simulink model "unrolled_pipelined_parallel"  (R2015b)
settings: Solver=FixedStepDiscrete  SolverMode=SingleTasking  StartTime=0.0  StopTime=10.0  RelTol=1e-3
undefined symbols (not defined in the file or in its folder): a, b
libraries: shlslibv1 x8781
(part 1 of 32)
settings Model: synDspstartup=OK  Creator=hchempat  LastModifiedBy=hchempat
settings DataIOCC: SaveOutput=off  SignalLogging=off  SaveTime=off
settings OptimizationCC: DefaultParameterBehavior=Inlined
settings DebuggingCC: AlgebraicLoopMsg=error  InheritedTsInSrcMsg=none

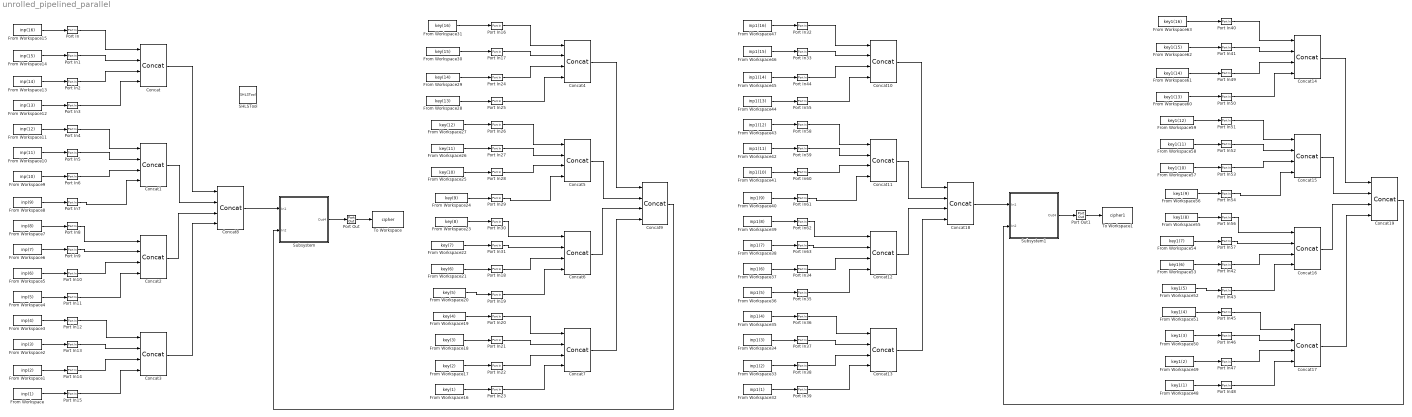
== system unrolled_pipelined_parallel ==
  Concat{,1..19} (20 alike) : shlslibv1/Signal Operations/Concat  syn_in_nb=4  syn_out_f=Automatic  syn_out_wl=16  syn_out_fl=8  syn_out_dt=signed  syn_en_se=off  synBlockType=primitive  synLatency=0  synBlockId=8
  From Workspace : FromWorkspace  VariableName=inp(1)
  From Workspace1 : FromWorkspace  VariableName=inp(2)
  From Workspace10 : FromWorkspace  VariableName=inp(11)
  From Workspace11 : FromWorkspace  VariableName=inp(12)
  From Workspace12 : FromWorkspace  VariableName=inp(13)
  From Workspace13 : FromWorkspace  VariableName=inp(14)
  From Workspace14 : FromWorkspace  VariableName=inp(15)
  From Workspace15 : FromWorkspace  VariableName=inp(16)
  From Workspace16 : FromWorkspace  VariableName=key(1)
  From Workspace17 : FromWorkspace  VariableName=key(2)
  From Workspace18 : FromWorkspace  VariableName=key(3)
  From Workspace19 : FromWorkspace  VariableName=key(4)
  From Workspace2 : FromWorkspace  VariableName=inp(3)
  From Workspace20 : FromWorkspace  VariableName=key(5)
  From Workspace21 : FromWorkspace  VariableName=key(6)
  From Workspace22 : FromWorkspace  VariableName=key(7)
  From Workspace23 : FromWorkspace  VariableName=key(8)
  From Workspace24 : FromWorkspace  VariableName=key(9)
  From Workspace25 : FromWorkspace  VariableName=key(10)
  From Workspace26 : FromWorkspace  VariableName=key(11)
  From Workspace27 : FromWorkspace  VariableName=key(12)
  From Workspace28 : FromWorkspace  VariableName=key(13)
  From Workspace29 : FromWorkspace  VariableName=key(14)
  From Workspace3 : FromWorkspace  VariableName=inp(4)
  From Workspace30 : FromWorkspace  VariableName=key(15)
  From Workspace31 : FromWorkspace  VariableName=key(16)
  From Workspace32 : FromWorkspace  VariableName=inp1(1)
  From Workspace33 : FromWorkspace  VariableName=inp1(2)
  From Workspace34 : FromWorkspace  VariableName=inp1(3)
  From Workspace35 : FromWorkspace  VariableName=inp1(4)
  From Workspace36 : FromWorkspace  VariableName=inp1(5)
  From Workspace37 : FromWorkspace  VariableName=inp1(6)
  From Workspace38 : FromWorkspace  VariableName=inp1(7)
  From Workspace39 : FromWorkspace  VariableName=inp1(8)
  From Workspace4 : FromWorkspace  VariableName=inp(5)
  From Workspace40 : FromWorkspace  VariableName=inp1(9)
  From Workspace41 : FromWorkspace  VariableName=inp1(10)
  From Workspace42 : FromWorkspace  VariableName=inp1(11)
  From Workspace43 : FromWorkspace  VariableName=inp1(12)
  From Workspace44 : FromWorkspace  VariableName=inp1(13)
  From Workspace45 : FromWorkspace  VariableName=inp1(14)
  From Workspace46 : FromWorkspace  VariableName=inp1(15)
  From Workspace47 : FromWorkspace  VariableName=inp1(16)
  From Workspace48 : FromWorkspace  VariableName=key1(1)
  From Workspace49 : FromWorkspace  VariableName=key1(2)
  From Workspace5 : FromWorkspace  VariableName=inp(6)
  From Workspace50 : FromWorkspace  VariableName=key1(3)
  From Workspace51 : FromWorkspace  VariableName=key1(4)
  From Workspace52 : FromWorkspace  VariableName=key1(5)
  From Workspace53 : FromWorkspace  VariableName=key1(6)
  From Workspace54 : FromWorkspace  VariableName=key1(7)
  From Workspace55 : FromWorkspace  VariableName=key1(8)
  From Workspace56 : FromWorkspace  VariableName=key1(9)
  From Workspace57 : FromWorkspace  VariableName=key1(10)
  From Workspace58 : FromWorkspace  VariableName=key1(11)
  From Workspace59 : FromWorkspace  VariableName=key1(12)
  From Workspace6 : FromWorkspace  VariableName=inp(7)
  From Workspace60 : FromWorkspace  VariableName=key1(13)
  From Workspace61 : FromWorkspace  VariableName=key1(14)
  From Workspace62 : FromWorkspace  VariableName=key1(15)
  From Workspace63 : FromWorkspace  VariableName=key1(16)
  From Workspace7 : FromWorkspace  VariableName=inp(8)
  From Workspace8 : FromWorkspace  VariableName=inp(9)
  From Workspace9 : FromWorkspace  VariableName=inp(10)
  Port In{,1..63} (64 alike) : shlslibv1/Ports & Subsystems/Port In  syn_out_wl=8  syn_out_fl=0  syn_out_dt=unsigned  syn_out_st=ts  syn_capture=on  syn_register=on  syn_out_sat=off  syn_out_rnd=on  synBlockType=port  synLatency=1  synBlockId=0
  Port Out : shlslibv1/Ports & Subsystems/Port Out  syn_capture=on  syn_register=on  synBlockType=port  synLatency=1  synBlockId=1
  Port Out1 : shlslibv1/Ports & Subsystems/Port Out  syn_capture=on  syn_register=on  synBlockType=port  synLatency=1  synBlockId=1
  SHLSTool : shlslibv1/SHLSTool  synBlockType=tool  syn_dsp_mode=FPGA
  Subsystem : Subsystem
  Subsystem1 : Subsystem
  To Workspace : ToWorkspace  VariableName=cipher  SaveFormat=Structure With Time  SampleTime=-1
  To Workspace1 : ToWorkspace  VariableName=cipher1  SaveFormat=Structure With Time  SampleTime=-1
  wires:
  From Workspace15/1 -> Port In/1
  From Workspace14/1 -> Port In1/1
  From Workspace12/1 -> Port In3/1
  From Workspace13/1 -> Port In2/1
  From Workspace11/1 -> Port In4/1
  From Workspace10/1 -> Port In5/1
  From Workspace9/1 -> Port In6/1
  From Workspace8/1 -> Port In7/1
  From Workspace7/1 -> Port In8/1
  From Workspace6/1 -> Port In9/1
  From Workspace5/1 -> Port In10/1
  From Workspace4/1 -> Port In11/1
  From Workspace3/1 -> Port In12/1
  From Workspace2/1 -> Port In13/1
  From Workspace1/1 -> Port In14/1
  From Workspace/1 -> Port In15/1
  Port In2/1 -> Concat/3
  Port In1/1 -> Concat/2
  Port In/1 -> Concat/1
  Port In3/1 -> Concat/4
  Port In6/1 -> Concat1/3
  Port In5/1 -> Concat1/2
  Port In4/1 -> Concat1/1
  Port In7/1 -> Concat1/4
  Port In10/1 -> Concat2/3
  Port In9/1 -> Concat2/2
  Port In8/1 -> Concat2/1
  Port In11/1 -> Concat2/4
  Port In14/1 -> Concat3/3
  Port In13/1 -> Concat3/2
  Port In15/1 -> Concat3/4
  Port In12/1 -> Concat3/1
  From Workspace22/1 -> Port In31/1
  From Workspace21/1 -> Port In18/1
  From Workspace20/1 -> Port In19/1
  From Workspace18/1 -> Port In21/1
  From Workspace17/1 -> Port In22/1
  From Workspace16/1 -> Port In23/1
  Port In24/1 -> Concat4/3
  Port In17/1 -> Concat4/2
  Port In16/1 -> Concat4/1
  Port In25/1 -> Concat4/4
  Port In28/1 -> Concat5/3
  Port In27/1 -> Concat5/2
  Port In26/1 -> Concat5/1
  Port In29/1 -> Concat5/4
  Port In18/1 -> Concat6/3
  Port In31/1 -> Concat6/2
  Port In30/1 -> Concat6/1
  Port In19/1 -> Concat6/4
  Port In22/1 -> Concat7/3
  Port In21/1 -> Concat7/2
  Port In23/1 -> Concat7/4
  Port In20/1 -> Concat7/1
  Concat/1 -> Concat8/1
  Concat1/1 -> Concat8/2
  Concat2/1 -> Concat8/3
  Concat3/1 -> Concat8/4
  Concat4/1 -> Concat9/1
  Concat5/1 -> Concat9/2
  Concat6/1 -> Concat9/3
  Concat7/1 -> Concat9/4
  Port Out/1 -> To Workspace/1
  Concat8/1 -> Subsystem/1(In1)
  Concat9/1 -> Subsystem/2(In2)
  Subsystem/1(Out4) -> Port Out/1
  From Workspace19/1 -> Port In20/1
  From Workspace23/1 -> Port In30/1
  From Workspace24/1 -> Port In29/1
  From Workspace25/1 -> Port In28/1
  From Workspace27/1 -> Port In26/1
  From Workspace28/1 -> Port In25/1
  From Workspace29/1 -> Port In24/1
  From Workspace30/1 -> Port In17/1
  From Workspace31/1 -> Port In16/1
  From Workspace26/1 -> Port In27/1
  From Workspace47/1 -> Port In32/1
  From Workspace46/1 -> Port In33/1
  From Workspace44/1 -> Port In55/1
  From Workspace45/1 -> Port In44/1
  From Workspace43/1 -> Port In58/1
  From Workspace42/1 -> Port In59/1
  From Workspace41/1 -> Port In60/1
  From Workspace40/1 -> Port In61/1
  From Workspace39/1 -> Port In62/1
  From Workspace38/1 -> Port In63/1
  From Workspace37/1 -> Port In34/1
  From Workspace36/1 -> Port In35/1
  From Workspace35/1 -> Port In36/1
  From Workspace34/1 -> Port In37/1
  From Workspace33/1 -> Port In38/1
  From Workspace32/1 -> Port In39/1
  Port In44/1 -> Concat10/3
  Port In33/1 -> Concat10/2
  Port In32/1 -> Concat10/1
  Port In55/1 -> Concat10/4
  Port In60/1 -> Concat11/3
  Port In59/1 -> Concat11/2
  Port In58/1 -> Concat11/1
  Port In61/1 -> Concat11/4
  Port In34/1 -> Concat12/3
  Port In63/1 -> Concat12/2
  Port In62/1 -> Concat12/1
  Port In35/1 -> Concat12/4
  Port In38/1 -> Concat13/3
  Port In37/1 -> Concat13/2
  Port In39/1 -> Concat13/4
  Port In36/1 -> Concat13/1
  From Workspace54/1 -> Port In57/1
  From Workspace53/1 -> Port In42/1
  From Workspace52/1 -> Port In43/1
  From Workspace50/1 -> Port In46/1
  From Workspace49/1 -> Port In47/1
  From Workspace48/1 -> Port In48/1
  Port In49/1 -> Concat14/3
  Port In41/1 -> Concat14/2
  Port In40/1 -> Concat14/1
  Port In50/1 -> Concat14/4
  Port In53/1 -> Concat15/3
  Port In52/1 -> Concat15/2
  Port In51/1 -> Concat15/1
  Port In54/1 -> Concat15/4
  Port In42/1 -> Concat16/3
  Port In57/1 -> Concat16/2
  Port In56/1 -> Concat16/1
  Port In43/1 -> Concat16/4
  Port In47/1 -> Concat17/3
  Port In46/1 -> Concat17/2
  Port In48/1 -> Concat17/4
  Port In45/1 -> Concat17/1
  Concat10/1 -> Concat18/1
  Concat11/1 -> Concat18/2
  Concat12/1 -> Concat18/3
  Concat13/1 -> Concat18/4
  Concat14/1 -> Concat19/1
  Concat15/1 -> Concat19/2
  Concat16/1 -> Concat19/3
  Concat17/1 -> Concat19/4
  Port Out1/1 -> To Workspace1/1
  Concat18/1 -> Subsystem1/1(In1)
  Concat19/1 -> Subsystem1/2(In2)
  Subsystem1/1(Out4) -> Port Out1/1
  From Workspace51/1 -> Port In45/1
  From Workspace55/1 -> Port In56/1
  From Workspace56/1 -> Port In54/1
  From Workspace57/1 -> Port In53/1
  From Workspace59/1 -> Port In51/1
  From Workspace60/1 -> Port In50/1
  From Workspace61/1 -> Port In49/1
  From Workspace62/1 -> Port In41/1
  From Workspace63/1 -> Port In40/1
  From Workspace58/1 -> Port In52/1

== system unrolled_pipelined_parallel/Subsystem ==
  In1 : Inport
  In2 : Inport  Port=2
  Concat : shlslibv1/Signal Operations/Concat  syn_in_nb=4  syn_out_f=Automatic  syn_out_wl=16  syn_out_fl=8  syn_out_dt=signed  syn_en_se=off  synBlockType=primitive  synLatency=0  synBlockId=8
  FINALROUND : Subsystem
  Register{1..50} (50 alike) : shlslibv1/Memories/Register  syn_delay_val=1  syn_rst_val=All zeros  syn_rst_vec=5  syn_rst_port=off  syn_en_port=off  synBlockType=custom  synLatency=1
  Subsystem : Subsystem
  Subsystem1 : Subsystem
  Subsystem2 : Subsystem
  Subsystem3 : Subsystem
  Subsystem4 : Subsystem
  Subsystem5 : Subsystem
  Subsystem6 : Subsystem
  Subsystem7 : Subsystem
  Subsystem8 : Subsystem
  Subsystem9 : Subsystem
  Out4 : Outport
  wires:
  FINALROUND/4(Out4) -> Concat/4
  FINALROUND/3(Out3) -> Concat/3
  FINALROUND/2(Out2) -> Concat/2
  FINALROUND/1(Out1) -> Concat/1
  In2/1 -> Register46/1, Subsystem/2(In2)
  In1/1 -> Subsystem/1(In1)
  Concat/1 -> Out4/1
  Subsystem1/5(Out5) -> Register5/1
  Register5/1 -> Subsystem2/5(In5)
  Subsystem1/2(Out2) -> Register2/1
  Subsystem1/3(Out3) -> Register3/1
  Subsystem1/4(Out4) -> Register4/1
  Subsystem1/1(Out1) -> Register1/1
  Register1/1 -> Subsystem2/1(In1)
  Register2/1 -> Subsystem2/2(In2)
  Register3/1 -> Subsystem2/3(In3)
  Register4/1 -> Subsystem2/4(In4)
  Subsystem2/5(Out5) -> Register10/1
  Subsystem2/2(Out2) -> Register7/1
  Subsystem2/3(Out3) -> Register8/1
  Subsystem2/4(Out4) -> Register9/1
  Subsystem2/1(Out1) -> Register6/1
  Register8/1 -> Subsystem3/3(In3)
  Register9/1 -> Subsystem3/4(In4)
  Register7/1 -> Subsystem3/2(In2)
  Register6/1 -> Subsystem3/1(In1)
  Register10/1 -> Subsystem3/5(In5)
  Subsystem3/5(Out5) -> Register11/1
  Subsystem3/2(Out2) -> Register13/1
  Subsystem3/3(Out3) -> Register14/1
  Subsystem3/4(Out4) -> Register15/1
  Subsystem3/1(Out1) -> Register12/1
  Register14/1 -> Subsystem4/3(In3)
  Register15/1 -> Subsystem4/4(In4)
  Register13/1 -> Subsystem4/2(In2)
  Register12/1 -> Subsystem4/1(In1)
  Register11/1 -> Subsystem4/5(In5)
  Subsystem4/5(Out5) -> Register16/1
  Subsystem4/2(Out2) -> Register18/1
  Subsystem4/3(Out3) -> Register19/1
  Subsystem4/4(Out4) -> Register20/1
  Subsystem4/1(Out1) -> Register17/1
  Register19/1 -> Subsystem5/3(In3)
  Register20/1 -> Subsystem5/4(In4)
  Register18/1 -> Subsystem5/2(In2)
  Register17/1 -> Subsystem5/1(In1)
  Register16/1 -> Subsystem5/5(In5)
  Subsystem5/5(Out5) -> Register21/1
  Subsystem5/2(Out2) -> Register23/1
  Subsystem5/3(Out3) -> Register24/1
  Subsystem5/4(Out4) -> Register25/1
  Subsystem5/1(Out1) -> Register22/1
  Register24/1 -> Subsystem6/3(In3)
  Register25/1 -> Subsystem6/4(In4)
  Register23/1 -> Subsystem6/2(In2)
  Register22/1 -> Subsystem6/1(In1)
  Register21/1 -> Subsystem6/5(In5)
  Subsystem6/5(Out5) -> Register26/1
  Subsystem6/2(Out2) -> Register28/1
  Subsystem6/3(Out3) -> Register29/1
  Subsystem6/4(Out4) -> Register30/1
  Subsystem6/1(Out1) -> Register27/1
  Register29/1 -> Subsystem7/3(In3)
  Register30/1 -> Subsystem7/4(In4)
  Register28/1 -> Subsystem7/2(In2)
  Register27/1 -> Subsystem7/1(In1)
  Register26/1 -> Subsystem7/5(In5)
  Subsystem7/5(Out5) -> Register31/1
  Subsystem7/2(Out2) -> Register33/1
  Subsystem7/3(Out3) -> Register34/1
  Subsystem7/4(Out4) -> Register35/1
  Subsystem7/1(Out1) -> Register32/1
  Register34/1 -> Subsystem8/3(In3)
  Register35/1 -> Subsystem8/4(In4)
  Register33/1 -> Subsystem8/2(In2)
  Register32/1 -> Subsystem8/1(In1)
  Register31/1 -> Subsystem8/5(In5)
  Subsystem8/5(Out5) -> Register36/1
  Subsystem8/2(Out2) -> Register38/1
  Subsystem8/3(Out3) -> Register39/1
  Subsystem8/4(Out4) -> Register40/1
  Subsystem8/1(Out1) -> Register37/1
  Register39/1 -> Subsystem9/3(In3)
  Register40/1 -> Subsystem9/4(In4)
  Register38/1 -> Subsystem9/2(In2)
  Register37/1 -> Subsystem9/1(In1)
  Register36/1 -> Subsystem9/5(In5)
  Subsystem9/5(Out5) -> Register41/1
  Subsystem9/2(Out2) -> Register43/1
  Subsystem9/3(Out3) -> Register44/1
  Subsystem9/4(Out4) -> Register45/1
  Subsystem9/1(Out1) -> Register42/1
  Register44/1 -> FINALROUND/3(In3)
  Register45/1 -> FINALROUND/4(In4)
  Register43/1 -> FINALROUND/2(In2)
  Register42/1 -> FINALROUND/1(In1)
  Register41/1 -> FINALROUND/5(In5)
  Register46/1 -> Subsystem1/5(In5)
  Subsystem/4(Out4) -> Register47/1
  Register47/1 -> Subsystem1/4(In4)
  Subsystem/1(Out1) -> Register50/1
  Register50/1 -> Subsystem1/1(In1)
  Subsystem/2(Out2) -> Register49/1
  Register49/1 -> Subsystem1/2(In2)
  Subsystem/3(Out3) -> Register48/1
  Register48/1 -> Subsystem1/3(In3)

== system unrolled_pipelined_parallel/Subsystem1 ==
  In1 : Inport
  In2 : Inport  Port=2
  Concat : shlslibv1/Signal Operations/Concat  syn_in_nb=4  syn_out_f=Automatic  syn_out_wl=16  syn_out_fl=8  syn_out_dt=signed  syn_en_se=off  synBlockType=primitive  synLatency=0  synBlockId=8
  FINALROUND : Subsystem
  Register{1..50} (50 alike) : shlslibv1/Memories/Register  syn_delay_val=1  syn_rst_val=All zeros  syn_rst_vec=5  syn_rst_port=off  syn_en_port=off  synBlockType=custom  synLatency=1
  Subsystem : Subsystem
  Subsystem1 : Subsystem
  Subsystem2 : Subsystem
  Subsystem3 : Subsystem
  Subsystem4 : Subsystem
  Subsystem5 : Subsystem
  Subsystem6 : Subsystem
  Subsystem7 : Subsystem
  Subsystem8 : Subsystem
  Subsystem9 : Subsystem
  Out4 : Outport
  wires:
  FINALROUND/4(Out4) -> Concat/4
  FINALROUND/3(Out3) -> Concat/3
  FINALROUND/2(Out2) -> Concat/2
  FINALROUND/1(Out1) -> Concat/1
  In2/1 -> Register46/1, Subsystem/2(In2)
  In1/1 -> Subsystem/1(In1)
  Concat/1 -> Out4/1
  Subsystem1/5(Out5) -> Register5/1
  Register5/1 -> Subsystem2/5(In5)
  Subsystem1/2(Out2) -> Register2/1
  Subsystem1/3(Out3) -> Register3/1
  Subsystem1/4(Out4) -> Register4/1
  Subsystem1/1(Out1) -> Register1/1
  Register1/1 -> Subsystem2/1(In1)
  Register2/1 -> Subsystem2/2(In2)
  Register3/1 -> Subsystem2/3(In3)
  Register4/1 -> Subsystem2/4(In4)
  Subsystem2/5(Out5) -> Register10/1
  Subsystem2/2(Out2) -> Register7/1
  Subsystem2/3(Out3) -> Register8/1
  Subsystem2/4(Out4) -> Register9/1
  Subsystem2/1(Out1) -> Register6/1
  Register8/1 -> Subsystem3/3(In3)
  Register9/1 -> Subsystem3/4(In4)
  Register7/1 -> Subsystem3/2(In2)
  Register6/1 -> Subsystem3/1(In1)
  Register10/1 -> Subsystem3/5(In5)
  Subsystem3/5(Out5) -> Register11/1
  Subsystem3/2(Out2) -> Register13/1
  Subsystem3/3(Out3) -> Register14/1
  Subsystem3/4(Out4) -> Register15/1
  Subsystem3/1(Out1) -> Register12/1
  Register14/1 -> Subsystem4/3(In3)
  Register15/1 -> Subsystem4/4(In4)
  Register13/1 -> Subsystem4/2(In2)
  Register12/1 -> Subsystem4/1(In1)
  Register11/1 -> Subsystem4/5(In5)
  Subsystem4/5(Out5) -> Register16/1
  Subsystem4/2(Out2) -> Register18/1
  Subsystem4/3(Out3) -> Register19/1
  Subsystem4/4(Out4) -> Register20/1
  Subsystem4/1(Out1) -> Register17/1
  Register19/1 -> Subsystem5/3(In3)
  Register20/1 -> Subsystem5/4(In4)
  Register18/1 -> Subsystem5/2(In2)
  Register17/1 -> Subsystem5/1(In1)
  Register16/1 -> Subsystem5/5(In5)
  Subsystem5/5(Out5) -> Register21/1
  Subsystem5/2(Out2) -> Register23/1
  Subsystem5/3(Out3) -> Register24/1
  Subsystem5/4(Out4) -> Register25/1
  Subsystem5/1(Out1) -> Register22/1
  Register24/1 -> Subsystem6/3(In3)
  Register25/1 -> Subsystem6/4(In4)
  Register23/1 -> Subsystem6/2(In2)
  Register22/1 -> Subsystem6/1(In1)
  Register21/1 -> Subsystem6/5(In5)
  Subsystem6/5(Out5) -> Register26/1
  Subsystem6/2(Out2) -> Register28/1
  Subsystem6/3(Out3) -> Register29/1
  Subsystem6/4(Out4) -> Register30/1
  Subsystem6/1(Out1) -> Register27/1
  Register29/1 -> Subsystem7/3(In3)
  Register30/1 -> Subsystem7/4(In4)
  Register28/1 -> Subsystem7/2(In2)
  Register27/1 -> Subsystem7/1(In1)
  Register26/1 -> Subsystem7/5(In5)
  Subsystem7/5(Out5) -> Register31/1
  Subsystem7/2(Out2) -> Register33/1
  Subsystem7/3(Out3) -> Register34/1
  Subsystem7/4(Out4) -> Register35/1
  Subsystem7/1(Out1) -> Register32/1
  Register34/1 -> Subsystem8/3(In3)
  Register35/1 -> Subsystem8/4(In4)
  Register33/1 -> Subsystem8/2(In2)
  Register32/1 -> Subsystem8/1(In1)
  Register31/1 -> Subsystem8/5(In5)
  Subsystem8/5(Out5) -> Register36/1
  Subsystem8/2(Out2) -> Register38/1
  Subsystem8/3(Out3) -> Register39/1
  Subsystem8/4(Out4) -> Register40/1
  Subsystem8/1(Out1) -> Register37/1
  Register39/1 -> Subsystem9/3(In3)
  Register40/1 -> Subsystem9/4(In4)
  Register38/1 -> Subsystem9/2(In2)
  Register37/1 -> Subsystem9/1(In1)
  Register36/1 -> Subsystem9/5(In5)
  Subsystem9/5(Out5) -> Register41/1
  Subsystem9/2(Out2) -> Register43/1
  Subsystem9/3(Out3) -> Register44/1
  Subsystem9/4(Out4) -> Register45/1
  Subsystem9/1(Out1) -> Register42/1
  Register44/1 -> FINALROUND/3(In3)
  Register45/1 -> FINALROUND/4(In4)
  Register43/1 -> FINALROUND/2(In2)
  Register42/1 -> FINALROUND/1(In1)
  Register41/1 -> FINALROUND/5(In5)
  Register46/1 -> Subsystem1/5(In5)
  Subsystem/4(Out4) -> Register47/1
  Register47/1 -> Subsystem1/4(In4)
  Subsystem/1(Out1) -> Register50/1
  Register50/1 -> Subsystem1/1(In1)
  Subsystem/2(Out2) -> Register49/1
  Register49/1 -> Subsystem1/2(In2)
  Subsystem/3(Out3) -> Register48/1
  Register48/1 -> Subsystem1/3(In3)

== system unrolled_pipelined_parallel/Subsystem/FINALROUND ==
  In1 : Inport
  In2 : Inport  Port=2
  In3 : Inport  Port=3
  In4 : Inport  Port=4
  In5 : Inport  Port=5
  ADD ROUND KEY : Subsystem
  KEYEXPANSION : Subsystem
  SB_rs_MIX_COLUMN : Subsystem
  Out1 : Outport
  Out2 : Outport  Port=2
  Out3 : Outport  Port=3
  Out4 : Outport  Port=4
  wires:
  SB_rs_MIX_COLUMN/1(Out1) -> ADD ROUND KEY/1(In1)
  KEYEXPANSION/1(Out1) -> ADD ROUND KEY/2(In2)
  In1/1 -> SB_rs_MIX_COLUMN/1(In1)
  In2/1 -> SB_rs_MIX_COLUMN/2(In2)
  In3/1 -> SB_rs_MIX_COLUMN/3(In3)
  In4/1 -> SB_rs_MIX_COLUMN/4(In4)
  In5/1 -> KEYEXPANSION/1(In1)
  ADD ROUND KEY/1(Out1) -> Out1/1
  ADD ROUND KEY/2(Out2) -> Out2/1
  ADD ROUND KEY/3(Out3) -> Out3/1
  ADD ROUND KEY/4(Out4) -> Out4/1

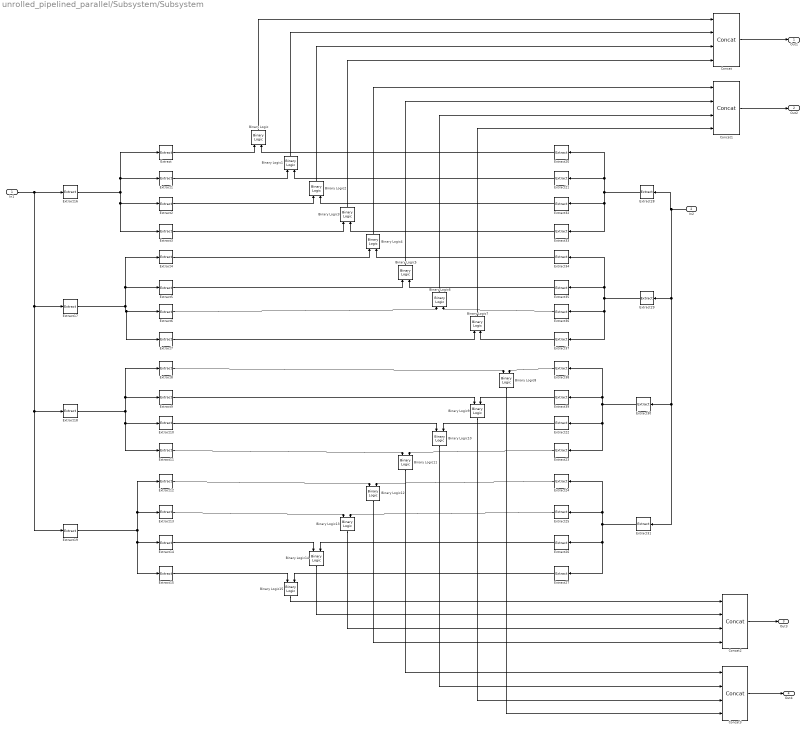
== system unrolled_pipelined_parallel/Subsystem/Subsystem ==
  In1 : Inport
  In2 : Inport  Port=2
  Binary Logic{,1..15} (16 alike) : shlslibv1/Math Functions/Binary Logic  syn_binlog_exp=a^b  synBlockType=primitive  synLatency=0  synBlockId=13
  Concat{,1..3} (4 alike) : shlslibv1/Signal Operations/Concat  syn_in_nb=4  syn_out_f=Automatic  syn_out_wl=16  syn_out_fl=8  syn_out_dt=signed  syn_en_se=off  synBlockType=primitive  synLatency=0  synBlockId=8
  Extract{,4,8,12,20,24,34,38} (8 alike) : shlslibv1/Signal Operations/Extract  syn_extract_vec=[24:31]  synBlockType=primitive  synLatency=0  synBlockId=17
  Extract{1,5,9,13,21,25,35,39} (8 alike) : shlslibv1/Signal Operations/Extract  syn_extract_vec=[16:23]  synBlockType=primitive  synLatency=0  synBlockId=17
  Extract{2,6,10,14,22,26,32,36} (8 alike) : shlslibv1/Signal Operations/Extract  syn_extract_vec=[8:15]  synBlockType=primitive  synLatency=0  synBlockId=17
  Extract{3,7,11,15,23,27,33,37} (8 alike) : shlslibv1/Signal Operations/Extract  syn_extract_vec=[0:7]  synBlockType=primitive  synLatency=0  synBlockId=17
  Extract16 : shlslibv1/Signal Operations/Extract  syn_extract_vec=[96:127]  synBlockType=primitive  synLatency=0  synBlockId=17
  Extract17 : shlslibv1/Signal Operations/Extract  syn_extract_vec=[64:95]  synBlockType=primitive  synLatency=0  synBlockId=17
  Extract18 : shlslibv1/Signal Operations/Extract  syn_extract_vec=[32:63]  synBlockType=primitive  synLatency=0  synBlockId=17
  Extract19 : shlslibv1/Signal Operations/Extract  syn_extract_vec=[0:31]  synBlockType=primitive  synLatency=0  synBlockId=17
  Extract28 : shlslibv1/Signal Operations/Extract  syn_extract_vec=[96:127]  synBlockType=primitive  synLatency=0  synBlockId=17
  Extract29 : shlslibv1/Signal Operations/Extract  syn_extract_vec=[64:95]  synBlockType=primitive  synLatency=0  synBlockId=17
  Extract30 : shlslibv1/Signal Operations/Extract  syn_extract_vec=[32:63]  synBlockType=primitive  synLatency=0  synBlockId=17
  Extract31 : shlslibv1/Signal Operations/Extract  syn_extract_vec=[0:31]  synBlockType=primitive  synLatency=0  synBlockId=17
  Out1 : Outport
  Out2 : Outport  Port=2
  Out3 : Outport  Port=3
  Out4 : Outport  Port=4
  wires:
  Extract16/1 -> Extract/1, Extract1/1, Extract2/1, Extract3/1
  Extract17/1 -> Extract6/1, Extract7/1, Extract4/1, Extract5/1
  Extract18/1 -> Extract9/1, Extract8/1, Extract10/1, Extract11/1
  Extract19/1 -> Extract12/1, Extract13/1, Extract15/1, Extract14/1
  In1/1 -> Extract19/1, Extract18/1, Extract17/1, Extract16/1
  In2/1 -> Extract31/1, Extract30/1, Extract29/1, Extract28/1
  Extract28/1 -> Extract21/1, Extract20/1, Extract33/1, Extract32/1
  Extract29/1 -> Extract35/1, Extract34/1, Extract36/1, Extract37/1
  Extract30/1 -> Extract23/1, Extract22/1, Extract38/1, Extract39/1
  Extract31/1 -> Extract24/1, Extract25/1, Extract27/1, Extract26/1
  Extract/1 -> Binary Logic/1
  Extract20/1 -> Binary Logic/2
  Extract1/1 -> Binary Logic1/1
  Extract21/1 -> Binary Logic1/2
  Extract2/1 -> Binary Logic2/1
  Extract32/1 -> Binary Logic2/2
  Extract3/1 -> Binary Logic3/1
  Extract33/1 -> Binary Logic3/2
  Extract4/1 -> Binary Logic4/1
  Extract34/1 -> Binary Logic4/2
  Extract5/1 -> Binary Logic5/1
  Extract35/1 -> Binary Logic5/2
  Extract6/1 -> Binary Logic6/1
  Extract36/1 -> Binary Logic6/2
  Extract7/1 -> Binary Logic7/1
  Extract37/1 -> Binary Logic7/2
  Extract8/1 -> Binary Logic8/1
  Extract38/1 -> Binary Logic8/2
  Extract9/1 -> Binary Logic9/1
  Extract39/1 -> Binary Logic9/2
  Extract22/1 -> Binary Logic10/2
  Extract10/1 -> Binary Logic10/1
  Extract23/1 -> Binary Logic11/2
  Extract11/1 -> Binary Logic11/1
  Extract12/1 -> Binary Logic12/1
  Extract24/1 -> Binary Logic12/2
  Extract13/1 -> Binary Logic13/1
  Extract25/1 -> Binary Logic13/2
  Extract14/1 -> Binary Logic14/1
  Extract26/1 -> Binary Logic14/2
  Extract15/1 -> Binary Logic15/1
  Extract27/1 -> Binary Logic15/2
  Binary Logic7/1 -> Concat1/4
  Binary Logic6/1 -> Concat1/3
  Binary Logic5/1 -> Concat1/2
  Binary Logic4/1 -> Concat1/1
  Binary Logic3/1 -> Concat/4
  Binary Logic2/1 -> Concat/3
  Binary Logic1/1 -> Concat/2
  Binary Logic/1 -> Concat/1
  Binary Logic15/1 -> Concat2/1
  Binary Logic14/1 -> Concat2/2
  Binary Logic13/1 -> Concat2/3
  Binary Logic12/1 -> Concat2/4
  Binary Logic11/1 -> Concat3/1
  Binary Logic10/1 -> Concat3/2
  Binary Logic9/1 -> Concat3/3
  Binary Logic8/1 -> Concat3/4
  Concat/1 -> Out1/1
  Concat1/1 -> Out2/1
  Concat2/1 -> Out3/1
  Concat3/1 -> Out4/1

== system unrolled_pipelined_parallel/Subsystem/Subsystem1 ==
  In1 : Inport
  In2 : Inport  Port=2
  In3 : Inport  Port=3
  In4 : Inport  Port=4
  In5 : Inport  Port=5
  ADD ROUND KEY : Subsystem
  KEYEXPANSION : Subsystem
  SB_rs_MIX_COLUMN : Subsystem
  Out1 : Outport
  Out2 : Outport  Port=2
  Out3 : Outport  Port=3
  Out4 : Outport  Port=4
  Out5 : Outport  Port=5
  wires:
  SB_rs_MIX_COLUMN/1(Out1) -> ADD ROUND KEY/1(In1)
  KEYEXPANSION/1(Out1) -> Out5/1, ADD ROUND KEY/2(In2)
  In1/1 -> SB_rs_MIX_COLUMN/1(In1)
  In2/1 -> SB_rs_MIX_COLUMN/2(In2)
  In3/1 -> SB_rs_MIX_COLUMN/3(In3)
  In4/1 -> SB_rs_MIX_COLUMN/4(In4)
  In5/1 -> KEYEXPANSION/1(In1)
  ADD ROUND KEY/1(Out1) -> Out1/1
  ADD ROUND KEY/2(Out2) -> Out2/1
  ADD ROUND KEY/3(Out3) -> Out3/1
  ADD ROUND KEY/4(Out4) -> Out4/1

== system unrolled_pipelined_parallel/Subsystem/Subsystem2 ==
  In1 : Inport
  In2 : Inport  Port=2
  In3 : Inport  Port=3
  In4 : Inport  Port=4
  In5 : Inport  Port=5
  ADD ROUND KEY : Subsystem
  KEYEXPANSION : Subsystem
  SB_rs_MIX_COLUMN : Subsystem
  Out1 : Outport
  Out2 : Outport  Port=2
  Out3 : Outport  Port=3
  Out4 : Outport  Port=4
  Out5 : Outport  Port=5
  wires:
  SB_rs_MIX_COLUMN/1(Out1) -> ADD ROUND KEY/1(In1)
  KEYEXPANSION/1(Out1) -> Out5/1, ADD ROUND KEY/2(In2)
  In1/1 -> SB_rs_MIX_COLUMN/1(In1)
  In2/1 -> SB_rs_MIX_COLUMN/2(In2)
  In3/1 -> SB_rs_MIX_COLUMN/3(In3)
  In4/1 -> SB_rs_MIX_COLUMN/4(In4)
  In5/1 -> KEYEXPANSION/1(In1)
  ADD ROUND KEY/1(Out1) -> Out1/1
  ADD ROUND KEY/2(Out2) -> Out2/1
  ADD ROUND KEY/3(Out3) -> Out3/1
  ADD ROUND KEY/4(Out4) -> Out4/1

== system unrolled_pipelined_parallel/Subsystem/Subsystem3 ==
  In1 : Inport
  In2 : Inport  Port=2
  In3 : Inport  Port=3
  In4 : Inport  Port=4
  In5 : Inport  Port=5
  ADD ROUND KEY : Subsystem
  KEYEXPANSION : Subsystem
  SB_rs_MIX_COLUMN : Subsystem
  Out1 : Outport
  Out2 : Outport  Port=2
  Out3 : Outport  Port=3
  Out4 : Outport  Port=4
  Out5 : Outport  Port=5
  wires:
  SB_rs_MIX_COLUMN/1(Out1) -> ADD ROUND KEY/1(In1)
  KEYEXPANSION/1(Out1) -> Out5/1, ADD ROUND KEY/2(In2)
  In1/1 -> SB_rs_MIX_COLUMN/1(In1)
  In2/1 -> SB_rs_MIX_COLUMN/2(In2)
  In3/1 -> SB_rs_MIX_COLUMN/3(In3)
  In4/1 -> SB_rs_MIX_COLUMN/4(In4)
  In5/1 -> KEYEXPANSION/1(In1)
  ADD ROUND KEY/1(Out1) -> Out1/1
  ADD ROUND KEY/2(Out2) -> Out2/1
  ADD ROUND KEY/3(Out3) -> Out3/1
  ADD ROUND KEY/4(Out4) -> Out4/1

== system unrolled_pipelined_parallel/Subsystem/Subsystem4 ==
  In1 : Inport
  In2 : Inport  Port=2
  In3 : Inport  Port=3
  In4 : Inport  Port=4
  In5 : Inport  Port=5
  ADD ROUND KEY : Subsystem
  KEYEXPANSION : Subsystem
  SB_rs_MIX_COLUMN : Subsystem
  Out1 : Outport
  Out2 : Outport  Port=2
  Out3 : Outport  Port=3
  Out4 : Outport  Port=4
  Out5 : Outport  Port=5
  wires:
  SB_rs_MIX_COLUMN/1(Out1) -> ADD ROUND KEY/1(In1)
  KEYEXPANSION/1(Out1) -> Out5/1, ADD ROUND KEY/2(In2)
  In1/1 -> SB_rs_MIX_COLUMN/1(In1)
  In2/1 -> SB_rs_MIX_COLUMN/2(In2)
  In3/1 -> SB_rs_MIX_COLUMN/3(In3)
  In4/1 -> SB_rs_MIX_COLUMN/4(In4)
  In5/1 -> KEYEXPANSION/1(In1)
  ADD ROUND KEY/1(Out1) -> Out1/1
  ADD ROUND KEY/2(Out2) -> Out2/1
  ADD ROUND KEY/3(Out3) -> Out3/1
  ADD ROUND KEY/4(Out4) -> Out4/1

== system unrolled_pipelined_parallel/Subsystem/Subsystem5 ==
  In1 : Inport
  In2 : Inport  Port=2
  In3 : Inport  Port=3
  In4 : Inport  Port=4
  In5 : Inport  Port=5
  ADD ROUND KEY : Subsystem
  KEYEXPANSION : Subsystem
  SB_rs_MIX_COLUMN : Subsystem
  Out1 : Outport
  Out2 : Outport  Port=2
  Out3 : Outport  Port=3
  Out4 : Outport  Port=4
  Out5 : Outport  Port=5
  wires:
  SB_rs_MIX_COLUMN/1(Out1) -> ADD ROUND KEY/1(In1)
  KEYEXPANSION/1(Out1) -> Out5/1, ADD ROUND KEY/2(In2)
  In1/1 -> SB_rs_MIX_COLUMN/1(In1)
  In2/1 -> SB_rs_MIX_COLUMN/2(In2)
  In3/1 -> SB_rs_MIX_COLUMN/3(In3)
  In4/1 -> SB_rs_MIX_COLUMN/4(In4)
  In5/1 -> KEYEXPANSION/1(In1)
  ADD ROUND KEY/1(Out1) -> Out1/1
  ADD ROUND KEY/2(Out2) -> Out2/1
  ADD ROUND KEY/3(Out3) -> Out3/1
  ADD ROUND KEY/4(Out4) -> Out4/1

== system unrolled_pipelined_parallel/Subsystem/Subsystem6 ==
  In1 : Inport
  In2 : Inport  Port=2
  In3 : Inport  Port=3
  In4 : Inport  Port=4
  In5 : Inport  Port=5
  ADD ROUND KEY : Subsystem
  KEYEXPANSION : Subsystem
  SB_rs_MIX_COLUMN : Subsystem
  Out1 : Outport
  Out2 : Outport  Port=2
  Out3 : Outport  Port=3
  Out4 : Outport  Port=4
  Out5 : Outport  Port=5
  wires:
  SB_rs_MIX_COLUMN/1(Out1) -> ADD ROUND KEY/1(In1)
  KEYEXPANSION/1(Out1) -> Out5/1, ADD ROUND KEY/2(In2)
  In1/1 -> SB_rs_MIX_COLUMN/1(In1)
  In2/1 -> SB_rs_MIX_COLUMN/2(In2)
  In3/1 -> SB_rs_MIX_COLUMN/3(In3)
  In4/1 -> SB_rs_MIX_COLUMN/4(In4)
  In5/1 -> KEYEXPANSION/1(In1)
  ADD ROUND KEY/1(Out1) -> Out1/1
  ADD ROUND KEY/2(Out2) -> Out2/1
  ADD ROUND KEY/3(Out3) -> Out3/1
  ADD ROUND KEY/4(Out4) -> Out4/1

== system unrolled_pipelined_parallel/Subsystem/Subsystem7 ==
  In1 : Inport
  In2 : Inport  Port=2
  In3 : Inport  Port=3
  In4 : Inport  Port=4
  In5 : Inport  Port=5
  ADD ROUND KEY : Subsystem
  KEYEXPANSION : Subsystem
  SB_rs_MIX_COLUMN : Subsystem
  Out1 : Outport
  Out2 : Outport  Port=2
  Out3 : Outport  Port=3
  Out4 : Outport  Port=4
  Out5 : Outport  Port=5
  wires:
  SB_rs_MIX_COLUMN/1(Out1) -> ADD ROUND KEY/1(In1)
  KEYEXPANSION/1(Out1) -> Out5/1, ADD ROUND KEY/2(In2)
  In1/1 -> SB_rs_MIX_COLUMN/1(In1)
  In2/1 -> SB_rs_MIX_COLUMN/2(In2)
  In3/1 -> SB_rs_MIX_COLUMN/3(In3)
  In4/1 -> SB_rs_MIX_COLUMN/4(In4)
  In5/1 -> KEYEXPANSION/1(In1)
  ADD ROUND KEY/1(Out1) -> Out1/1
  ADD ROUND KEY/2(Out2) -> Out2/1
  ADD ROUND KEY/3(Out3) -> Out3/1
  ADD ROUND KEY/4(Out4) -> Out4/1

== system unrolled_pipelined_parallel/Subsystem/Subsystem8 ==
  In1 : Inport
  In2 : Inport  Port=2
  In3 : Inport  Port=3
  In4 : Inport  Port=4
  In5 : Inport  Port=5
  ADD ROUND KEY : Subsystem
  KEYEXPANSION : Subsystem
  SB_rs_MIX_COLUMN : Subsystem
  Out1 : Outport
  Out2 : Outport  Port=2
  Out3 : Outport  Port=3
  Out4 : Outport  Port=4
  Out5 : Outport  Port=5
  wires:
  SB_rs_MIX_COLUMN/1(Out1) -> ADD ROUND KEY/1(In1)
  KEYEXPANSION/1(Out1) -> Out5/1, ADD ROUND KEY/2(In2)
  In1/1 -> SB_rs_MIX_COLUMN/1(In1)
  In2/1 -> SB_rs_MIX_COLUMN/2(In2)
  In3/1 -> SB_rs_MIX_COLUMN/3(In3)
  In4/1 -> SB_rs_MIX_COLUMN/4(In4)
  In5/1 -> KEYEXPANSION/1(In1)
  ADD ROUND KEY/1(Out1) -> Out1/1
  ADD ROUND KEY/2(Out2) -> Out2/1
  ADD ROUND KEY/3(Out3) -> Out3/1
  ADD ROUND KEY/4(Out4) -> Out4/1

== system unrolled_pipelined_parallel/Subsystem/Subsystem9 ==
  In1 : Inport
  In2 : Inport  Port=2
  In3 : Inport  Port=3
  In4 : Inport  Port=4
  In5 : Inport  Port=5
  ADD ROUND KEY : Subsystem
  KEYEXPANSION : Subsystem
  SB_rs_MIX_COLUMN : Subsystem
  Out1 : Outport
  Out2 : Outport  Port=2
  Out3 : Outport  Port=3
  Out4 : Outport  Port=4
  Out5 : Outport  Port=5
  wires:
  SB_rs_MIX_COLUMN/1(Out1) -> ADD ROUND KEY/1(In1)
  KEYEXPANSION/1(Out1) -> Out5/1, ADD ROUND KEY/2(In2)
  In1/1 -> SB_rs_MIX_COLUMN/1(In1)
  In2/1 -> SB_rs_MIX_COLUMN/2(In2)
  In3/1 -> SB_rs_MIX_COLUMN/3(In3)
  In4/1 -> SB_rs_MIX_COLUMN/4(In4)
  In5/1 -> KEYEXPANSION/1(In1)
  ADD ROUND KEY/1(Out1) -> Out1/1
  ADD ROUND KEY/2(Out2) -> Out2/1
  ADD ROUND KEY/3(Out3) -> Out3/1
  ADD ROUND KEY/4(Out4) -> Out4/1

== system unrolled_pipelined_parallel/Subsystem1/FINALROUND ==
  In1 : Inport
  In2 : Inport  Port=2
  In3 : Inport  Port=3
  In4 : Inport  Port=4
  In5 : Inport  Port=5
  ADD ROUND KEY : Subsystem
  KEYEXPANSION : Subsystem
  SB_rs_MIX_COLUMN : Subsystem
  Out1 : Outport
  Out2 : Outport  Port=2
  Out3 : Outport  Port=3
  Out4 : Outport  Port=4
  wires:
  SB_rs_MIX_COLUMN/1(Out1) -> ADD ROUND KEY/1(In1)
  KEYEXPANSION/1(Out1) -> ADD ROUND KEY/2(In2)
  In1/1 -> SB_rs_MIX_COLUMN/1(In1)
  In2/1 -> SB_rs_MIX_COLUMN/2(In2)
  In3/1 -> SB_rs_MIX_COLUMN/3(In3)
  In4/1 -> SB_rs_MIX_COLUMN/4(In4)
  In5/1 -> KEYEXPANSION/1(In1)
  ADD ROUND KEY/1(Out1) -> Out1/1
  ADD ROUND KEY/2(Out2) -> Out2/1
  ADD ROUND KEY/3(Out3) -> Out3/1
  ADD ROUND KEY/4(Out4) -> Out4/1

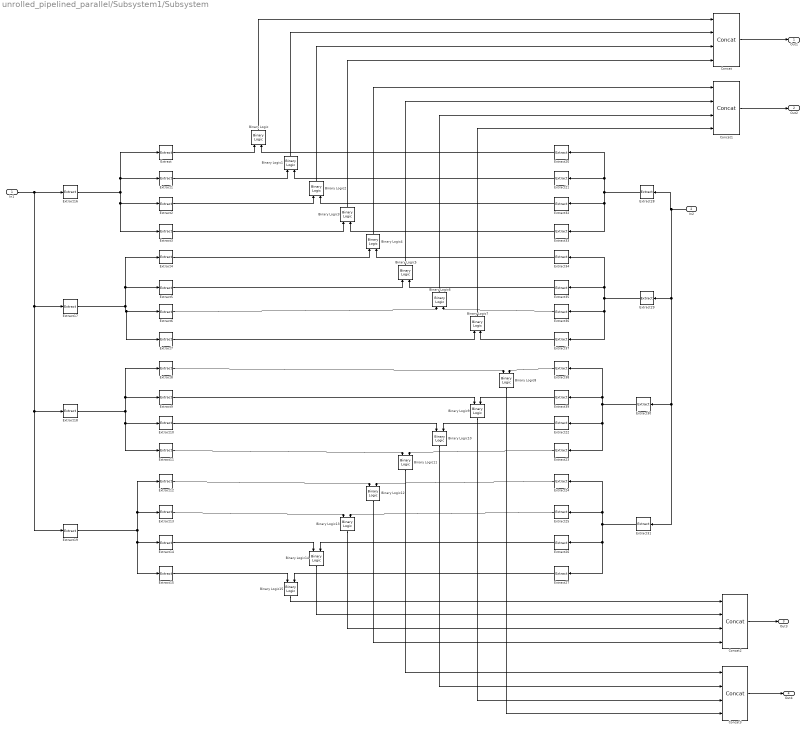
== system unrolled_pipelined_parallel/Subsystem1/Subsystem ==
  In1 : Inport
  In2 : Inport  Port=2
  Binary Logic{,1..15} (16 alike) : shlslibv1/Math Functions/Binary Logic  syn_binlog_exp=a^b  synBlockType=primitive  synLatency=0  synBlockId=13
  Concat{,1..3} (4 alike) : shlslibv1/Signal Operations/Concat  syn_in_nb=4  syn_out_f=Automatic  syn_out_wl=16  syn_out_fl=8  syn_out_dt=signed  syn_en_se=off  synBlockType=primitive  synLatency=0  synBlockId=8
  Extract{,4,8,12,20,24,34,38} (8 alike) : shlslibv1/Signal Operations/Extract  syn_extract_vec=[24:31]  synBlockType=primitive  synLatency=0  synBlockId=17
  Extract{1,5,9,13,21,25,35,39} (8 alike) : shlslibv1/Signal Operations/Extract  syn_extract_vec=[16:23]  synBlockType=primitive  synLatency=0  synBlockId=17
  Extract{2,6,10,14,22,26,32,36} (8 alike) : shlslibv1/Signal Operations/Extract  syn_extract_vec=[8:15]  synBlockType=primitive  synLatency=0  synBlockId=17
  Extract{3,7,11,15,23,27,33,37} (8 alike) : shlslibv1/Signal Operations/Extract  syn_extract_vec=[0:7]  synBlockType=primitive  synLatency=0  synBlockId=17
  Extract16 : shlslibv1/Signal Operations/Extract  syn_extract_vec=[96:127]  synBlockType=primitive  synLatency=0  synBlockId=17
  Extract17 : shlslibv1/Signal Operations/Extract  syn_extract_vec=[64:95]  synBlockType=primitive  synLatency=0  synBlockId=17
  Extract18 : shlslibv1/Signal Operations/Extract  syn_extract_vec=[32:63]  synBlockType=primitive  synLatency=0  synBlockId=17
  Extract19 : shlslibv1/Signal Operations/Extract  syn_extract_vec=[0:31]  synBlockType=primitive  synLatency=0  synBlockId=17
  Extract28 : shlslibv1/Signal Operations/Extract  syn_extract_vec=[96:127]  synBlockType=primitive  synLatency=0  synBlockId=17
  Extract29 : shlslibv1/Signal Operations/Extract  syn_extract_vec=[64:95]  synBlockType=primitive  synLatency=0  synBlockId=17
  Extract30 : shlslibv1/Signal Operations/Extract  syn_extract_vec=[32:63]  synBlockType=primitive  synLatency=0  synBlockId=17
  Extract31 : shlslibv1/Signal Operations/Extract  syn_extract_vec=[0:31]  synBlockType=primitive  synLatency=0  synBlockId=17
  Out1 : Outport
  Out2 : Outport  Port=2
  Out3 : Outport  Port=3
  Out4 : Outport  Port=4
  wires:
  Extract16/1 -> Extract/1, Extract1/1, Extract2/1, Extract3/1
  Extract17/1 -> Extract6/1, Extract7/1, Extract4/1, Extract5/1
  Extract18/1 -> Extract9/1, Extract8/1, Extract10/1, Extract11/1
  Extract19/1 -> Extract12/1, Extract13/1, Extract15/1, Extract14/1
  In1/1 -> Extract19/1, Extract18/1, Extract17/1, Extract16/1
  In2/1 -> Extract31/1, Extract30/1, Extract29/1, Extract28/1
  Extract28/1 -> Extract21/1, Extract20/1, Extract33/1, Extract32/1
  Extract29/1 -> Extract35/1, Extract34/1, Extract36/1, Extract37/1
  Extract30/1 -> Extract23/1, Extract22/1, Extract38/1, Extract39/1
  Extract31/1 -> Extract24/1, Extract25/1, Extract27/1, Extract26/1
  Extract/1 -> Binary Logic/1
  Extract20/1 -> Binary Logic/2
  Extract1/1 -> Binary Logic1/1
  Extract21/1 -> Binary Logic1/2
  Extract2/1 -> Binary Logic2/1
  Extract32/1 -> Binary Logic2/2
  Extract3/1 -> Binary Logic3/1
  Extract33/1 -> Binary Logic3/2
  Extract4/1 -> Binary Logic4/1
  Extract34/1 -> Binary Logic4/2
  Extract5/1 -> Binary Logic5/1
  Extract35/1 -> Binary Logic5/2
  Extract6/1 -> Binary Logic6/1
  Extract36/1 -> Binary Logic6/2
  Extract7/1 -> Binary Logic7/1
  Extract37/1 -> Binary Logic7/2
  Extract8/1 -> Binary Logic8/1
  Extract38/1 -> Binary Logic8/2
  Extract9/1 -> Binary Logic9/1
  Extract39/1 -> Binary Logic9/2
  Extract22/1 -> Binary Logic10/2
  Extract10/1 -> Binary Logic10/1
  Extract23/1 -> Binary Logic11/2
  Extract11/1 -> Binary Logic11/1
  Extract12/1 -> Binary Logic12/1
  Extract24/1 -> Binary Logic12/2
  Extract13/1 -> Binary Logic13/1
  Extract25/1 -> Binary Logic13/2
  Extract14/1 -> Binary Logic14/1
  Extract26/1 -> Binary Logic14/2
  Extract15/1 -> Binary Logic15/1
  Extract27/1 -> Binary Logic15/2
  Binary Logic7/1 -> Concat1/4
  Binary Logic6/1 -> Concat1/3
  Binary Logic5/1 -> Concat1/2
  Binary Logic4/1 -> Concat1/1
  Binary Logic3/1 -> Concat/4
  Binary Logic2/1 -> Concat/3
  Binary Logic1/1 -> Concat/2
  Binary Logic/1 -> Concat/1
  Binary Logic15/1 -> Concat2/1
  Binary Logic14/1 -> Concat2/2
  Binary Logic13/1 -> Concat2/3
  Binary Logic12/1 -> Concat2/4
  Binary Logic11/1 -> Concat3/1
  Binary Logic10/1 -> Concat3/2
  Binary Logic9/1 -> Concat3/3
  Binary Logic8/1 -> Concat3/4
  Concat/1 -> Out1/1
  Concat1/1 -> Out2/1
  Concat2/1 -> Out3/1
  Concat3/1 -> Out4/1

== system unrolled_pipelined_parallel/Subsystem1/Subsystem1 ==
  In1 : Inport
  In2 : Inport  Port=2
  In3 : Inport  Port=3
  In4 : Inport  Port=4
  In5 : Inport  Port=5
  ADD ROUND KEY : Subsystem
  KEYEXPANSION : Subsystem
  SB_rs_MIX_COLUMN : Subsystem
  Out1 : Outport
  Out2 : Outport  Port=2
  Out3 : Outport  Port=3
  Out4 : Outport  Port=4
  Out5 : Outport  Port=5
  wires:
  SB_rs_MIX_COLUMN/1(Out1) -> ADD ROUND KEY/1(In1)
  KEYEXPANSION/1(Out1) -> Out5/1, ADD ROUND KEY/2(In2)
  In1/1 -> SB_rs_MIX_COLUMN/1(In1)
  In2/1 -> SB_rs_MIX_COLUMN/2(In2)
  In3/1 -> SB_rs_MIX_COLUMN/3(In3)
  In4/1 -> SB_rs_MIX_COLUMN/4(In4)
  In5/1 -> KEYEXPANSION/1(In1)
  ADD ROUND KEY/1(Out1) -> Out1/1
  ADD ROUND KEY/2(Out2) -> Out2/1
  ADD ROUND KEY/3(Out3) -> Out3/1
  ADD ROUND KEY/4(Out4) -> Out4/1

== system unrolled_pipelined_parallel/Subsystem1/Subsystem2 ==
  In1 : Inport
  In2 : Inport  Port=2
  In3 : Inport  Port=3
  In4 : Inport  Port=4
  In5 : Inport  Port=5
  ADD ROUND KEY : Subsystem
  KEYEXPANSION : Subsystem
  SB_rs_MIX_COLUMN : Subsystem
  Out1 : Outport
  Out2 : Outport  Port=2
  Out3 : Outport  Port=3
  Out4 : Outport  Port=4
  Out5 : Outport  Port=5
  wires:
  SB_rs_MIX_COLUMN/1(Out1) -> ADD ROUND KEY/1(In1)
  KEYEXPANSION/1(Out1) -> Out5/1, ADD ROUND KEY/2(In2)
  In1/1 -> SB_rs_MIX_COLUMN/1(In1)
  In2/1 -> SB_rs_MIX_COLUMN/2(In2)
  In3/1 -> SB_rs_MIX_COLUMN/3(In3)
  In4/1 -> SB_rs_MIX_COLUMN/4(In4)
  In5/1 -> KEYEXPANSION/1(In1)
  ADD ROUND KEY/1(Out1) -> Out1/1
  ADD ROUND KEY/2(Out2) -> Out2/1
  ADD ROUND KEY/3(Out3) -> Out3/1
  ADD ROUND KEY/4(Out4) -> Out4/1

== system unrolled_pipelined_parallel/Subsystem1/Subsystem3 ==
  In1 : Inport
  In2 : Inport  Port=2
  In3 : Inport  Port=3
  In4 : Inport  Port=4
  In5 : Inport  Port=5
  ADD ROUND KEY : Subsystem
  KEYEXPANSION : Subsystem
  SB_rs_MIX_COLUMN : Subsystem
  Out1 : Outport
  Out2 : Outport  Port=2
  Out3 : Outport  Port=3
  Out4 : Outport  Port=4
  Out5 : Outport  Port=5
  wires:
  SB_rs_MIX_COLUMN/1(Out1) -> ADD ROUND KEY/1(In1)
  KEYEXPANSION/1(Out1) -> Out5/1, ADD ROUND KEY/2(In2)
  In1/1 -> SB_rs_MIX_COLUMN/1(In1)
  In2/1 -> SB_rs_MIX_COLUMN/2(In2)
  In3/1 -> SB_rs_MIX_COLUMN/3(In3)
  In4/1 -> SB_rs_MIX_COLUMN/4(In4)
  In5/1 -> KEYEXPANSION/1(In1)
  ADD ROUND KEY/1(Out1) -> Out1/1
  ADD ROUND KEY/2(Out2) -> Out2/1
  ADD ROUND KEY/3(Out3) -> Out3/1
  ADD ROUND KEY/4(Out4) -> Out4/1

== system unrolled_pipelined_parallel/Subsystem1/Subsystem4 ==
  In1 : Inport
  In2 : Inport  Port=2
  In3 : Inport  Port=3
  In4 : Inport  Port=4
  In5 : Inport  Port=5
  ADD ROUND KEY : Subsystem
  KEYEXPANSION : Subsystem
  SB_rs_MIX_COLUMN : Subsystem
  Out1 : Outport
  Out2 : Outport  Port=2
  Out3 : Outport  Port=3
  Out4 : Outport  Port=4
  Out5 : Outport  Port=5
  wires:
  SB_rs_MIX_COLUMN/1(Out1) -> ADD ROUND KEY/1(In1)
  KEYEXPANSION/1(Out1) -> Out5/1, ADD ROUND KEY/2(In2)
  In1/1 -> SB_rs_MIX_COLUMN/1(In1)
  In2/1 -> SB_rs_MIX_COLUMN/2(In2)
  In3/1 -> SB_rs_MIX_COLUMN/3(In3)
  In4/1 -> SB_rs_MIX_COLUMN/4(In4)
  In5/1 -> KEYEXPANSION/1(In1)
  ADD ROUND KEY/1(Out1) -> Out1/1
  ADD ROUND KEY/2(Out2) -> Out2/1
  ADD ROUND KEY/3(Out3) -> Out3/1
  ADD ROUND KEY/4(Out4) -> Out4/1

== system unrolled_pipelined_parallel/Subsystem1/Subsystem5 ==
  In1 : Inport
  In2 : Inport  Port=2
  In3 : Inport  Port=3
  In4 : Inport  Port=4
  In5 : Inport  Port=5
  ADD ROUND KEY : Subsystem
  KEYEXPANSION : Subsystem
  SB_rs_MIX_COLUMN : Subsystem
  Out1 : Outport
  Out2 : Outport  Port=2
  Out3 : Outport  Port=3
  Out4 : Outport  Port=4
  Out5 : Outport  Port=5
  wires:
  SB_rs_MIX_COLUMN/1(Out1) -> ADD ROUND KEY/1(In1)
  KEYEXPANSION/1(Out1) -> Out5/1, ADD ROUND KEY/2(In2)
  In1/1 -> SB_rs_MIX_COLUMN/1(In1)
  In2/1 -> SB_rs_MIX_COLUMN/2(In2)
  In3/1 -> SB_rs_MIX_COLUMN/3(In3)
  In4/1 -> SB_rs_MIX_COLUMN/4(In4)
  In5/1 -> KEYEXPANSION/1(In1)
  ADD ROUND KEY/1(Out1) -> Out1/1
  ADD ROUND KEY/2(Out2) -> Out2/1
  ADD ROUND KEY/3(Out3) -> Out3/1
  ADD ROUND KEY/4(Out4) -> Out4/1

== system unrolled_pipelined_parallel/Subsystem1/Subsystem6 ==
  In1 : Inport
  In2 : Inport  Port=2
  In3 : Inport  Port=3
  In4 : Inport  Port=4
  In5 : Inport  Port=5
  ADD ROUND KEY : Subsystem
  KEYEXPANSION : Subsystem
  SB_rs_MIX_COLUMN : Subsystem
  Out1 : Outport
  Out2 : Outport  Port=2
  Out3 : Outport  Port=3
  Out4 : Outport  Port=4
  Out5 : Outport  Port=5
  wires:
  SB_rs_MIX_COLUMN/1(Out1) -> ADD ROUND KEY/1(In1)
  KEYEXPANSION/1(Out1) -> Out5/1, ADD ROUND KEY/2(In2)
  In1/1 -> SB_rs_MIX_COLUMN/1(In1)
  In2/1 -> SB_rs_MIX_COLUMN/2(In2)
  In3/1 -> SB_rs_MIX_COLUMN/3(In3)
  In4/1 -> SB_rs_MIX_COLUMN/4(In4)
  In5/1 -> KEYEXPANSION/1(In1)
  ADD ROUND KEY/1(Out1) -> Out1/1
  ADD ROUND KEY/2(Out2) -> Out2/1
  ADD ROUND KEY/3(Out3) -> Out3/1
  ADD ROUND KEY/4(Out4) -> Out4/1

== system unrolled_pipelined_parallel/Subsystem1/Subsystem7 ==
  In1 : Inport
  In2 : Inport  Port=2
  In3 : Inport  Port=3
  In4 : Inport  Port=4
  In5 : Inport  Port=5
  ADD ROUND KEY : Subsystem
  KEYEXPANSION : Subsystem
  SB_rs_MIX_COLUMN : Subsystem
  Out1 : Outport
  Out2 : Outport  Port=2
  Out3 : Outport  Port=3
  Out4 : Outport  Port=4
  Out5 : Outport  Port=5
  wires:
  SB_rs_MIX_COLUMN/1(Out1) -> ADD ROUND KEY/1(In1)
  KEYEXPANSION/1(Out1) -> Out5/1, ADD ROUND KEY/2(In2)
  In1/1 -> SB_rs_MIX_COLUMN/1(In1)
  In2/1 -> SB_rs_MIX_COLUMN/2(In2)
  In3/1 -> SB_rs_MIX_COLUMN/3(In3)
  In4/1 -> SB_rs_MIX_COLUMN/4(In4)
  In5/1 -> KEYEXPANSION/1(In1)
  ADD ROUND KEY/1(Out1) -> Out1/1
  ADD ROUND KEY/2(Out2) -> Out2/1
  ADD ROUND KEY/3(Out3) -> Out3/1
  ADD ROUND KEY/4(Out4) -> Out4/1

== system unrolled_pipelined_parallel/Subsystem1/Subsystem8 ==
  In1 : Inport
  In2 : Inport  Port=2
  In3 : Inport  Port=3
  In4 : Inport  Port=4
  In5 : Inport  Port=5
  ADD ROUND KEY : Subsystem
  KEYEXPANSION : Subsystem
  SB_rs_MIX_COLUMN : Subsystem
  Out1 : Outport
  Out2 : Outport  Port=2
  Out3 : Outport  Port=3
  Out4 : Outport  Port=4
  Out5 : Outport  Port=5
  wires:
  SB_rs_MIX_COLUMN/1(Out1) -> ADD ROUND KEY/1(In1)
  KEYEXPANSION/1(Out1) -> Out5/1, ADD ROUND KEY/2(In2)
  In1/1 -> SB_rs_MIX_COLUMN/1(In1)
  In2/1 -> SB_rs_MIX_COLUMN/2(In2)
  In3/1 -> SB_rs_MIX_COLUMN/3(In3)
  In4/1 -> SB_rs_MIX_COLUMN/4(In4)
  In5/1 -> KEYEXPANSION/1(In1)
  ADD ROUND KEY/1(Out1) -> Out1/1
  ADD ROUND KEY/2(Out2) -> Out2/1
  ADD ROUND KEY/3(Out3) -> Out3/1
  ADD ROUND KEY/4(Out4) -> Out4/1

== system unrolled_pipelined_parallel/Subsystem1/Subsystem9 ==
  In1 : Inport
  In2 : Inport  Port=2
  In3 : Inport  Port=3
  In4 : Inport  Port=4
  In5 : Inport  Port=5
  ADD ROUND KEY : Subsystem
  KEYEXPANSION : Subsystem
  SB_rs_MIX_COLUMN : Subsystem
  Out1 : Outport
  Out2 : Outport  Port=2
  Out3 : Outport  Port=3
  Out4 : Outport  Port=4
  Out5 : Outport  Port=5
  wires:
  SB_rs_MIX_COLUMN/1(Out1) -> ADD ROUND KEY/1(In1)
  KEYEXPANSION/1(Out1) -> Out5/1, ADD ROUND KEY/2(In2)
  In1/1 -> SB_rs_MIX_COLUMN/1(In1)
  In2/1 -> SB_rs_MIX_COLUMN/2(In2)
  In3/1 -> SB_rs_MIX_COLUMN/3(In3)
  In4/1 -> SB_rs_MIX_COLUMN/4(In4)
  In5/1 -> KEYEXPANSION/1(In1)
  ADD ROUND KEY/1(Out1) -> Out1/1
  ADD ROUND KEY/2(Out2) -> Out2/1
  ADD ROUND KEY/3(Out3) -> Out3/1
  ADD ROUND KEY/4(Out4) -> Out4/1

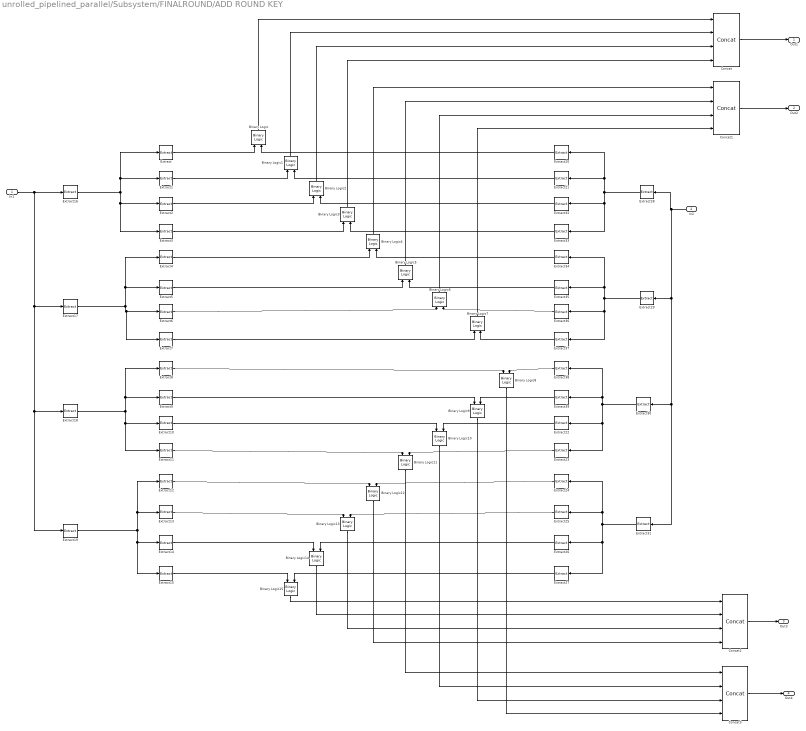
== system unrolled_pipelined_parallel/Subsystem/FINALROUND/ADD ROUND KEY ==
  In1 : Inport
  In2 : Inport  Port=2
  Binary Logic{,1..15} (16 alike) : shlslibv1/Math Functions/Binary Logic  syn_binlog_exp=a^b  synBlockType=primitive  synLatency=0  synBlockId=13
  Concat{,1..3} (4 alike) : shlslibv1/Signal Operations/Concat  syn_in_nb=4  syn_out_f=Automatic  syn_out_wl=16  syn_out_fl=8  syn_out_dt=signed  syn_en_se=off  synBlockType=primitive  synLatency=0  synBlockId=8
  Extract{,4,8,12,20,24,34,38} (8 alike) : shlslibv1/Signal Operations/Extract  syn_extract_vec=[24:31]  synBlockType=primitive  synLatency=0  synBlockId=17
  Extract{1,5,9,13,21,25,35,39} (8 alike) : shlslibv1/Signal Operations/Extract  syn_extract_vec=[16:23]  synBlockType=primitive  synLatency=0  synBlockId=17
  Extract{2,6,10,14,22,26,32,36} (8 alike) : shlslibv1/Signal Operations/Extract  syn_extract_vec=[8:15]  synBlockType=primitive  synLatency=0  synBlockId=17
  Extract{3,7,11,15,23,27,33,37} (8 alike) : shlslibv1/Signal Operations/Extract  syn_extract_vec=[0:7]  synBlockType=primitive  synLatency=0  synBlockId=17
  Extract16 : shlslibv1/Signal Operations/Extract  syn_extract_vec=[96:127]  synBlockType=primitive  synLatency=0  synBlockId=17
  Extract17 : shlslibv1/Signal Operations/Extract  syn_extract_vec=[64:95]  synBlockType=primitive  synLatency=0  synBlockId=17
  Extract18 : shlslibv1/Signal Operations/Extract  syn_extract_vec=[32:63]  synBlockType=primitive  synLatency=0  synBlockId=17
  Extract19 : shlslibv1/Signal Operations/Extract  syn_extract_vec=[0:31]  synBlockType=primitive  synLatency=0  synBlockId=17
  Extract28 : shlslibv1/Signal Operations/Extract  syn_extract_vec=[96:127]  synBlockType=primitive  synLatency=0  synBlockId=17
  Extract29 : shlslibv1/Signal Operations/Extract  syn_extract_vec=[64:95]  synBlockType=primitive  synLatency=0  synBlockId=17
  Extract30 : shlslibv1/Signal Operations/Extract  syn_extract_vec=[32:63]  synBlockType=primitive  synLatency=0  synBlockId=17
  Extract31 : shlslibv1/Signal Operations/Extract  syn_extract_vec=[0:31]  synBlockType=primitive  synLatency=0  synBlockId=17
  Out1 : Outport
  Out2 : Outport  Port=2
  Out3 : Outport  Port=3
  Out4 : Outport  Port=4
  wires:
  Extract16/1 -> Extract/1, Extract1/1, Extract2/1, Extract3/1
  Extract17/1 -> Extract6/1, Extract7/1, Extract4/1, Extract5/1
  Extract18/1 -> Extract9/1, Extract8/1, Extract10/1, Extract11/1
  Extract19/1 -> Extract12/1, Extract13/1, Extract15/1, Extract14/1
  In1/1 -> Extract19/1, Extract18/1, Extract17/1, Extract16/1
  In2/1 -> Extract31/1, Extract30/1, Extract29/1, Extract28/1
  Extract28/1 -> Extract21/1, Extract20/1, Extract33/1, Extract32/1
  Extract29/1 -> Extract35/1, Extract34/1, Extract36/1, Extract37/1
  Extract30/1 -> Extract23/1, Extract22/1, Extract38/1, Extract39/1
  Extract31/1 -> Extract24/1, Extract25/1, Extract27/1, Extract26/1
  Extract/1 -> Binary Logic/1
  Extract20/1 -> Binary Logic/2
  Extract1/1 -> Binary Logic1/1
  Extract21/1 -> Binary Logic1/2
  Extract2/1 -> Binary Logic2/1
  Extract32/1 -> Binary Logic2/2
  Extract3/1 -> Binary Logic3/1
  Extract33/1 -> Binary Logic3/2
  Extract4/1 -> Binary Logic4/1
  Extract34/1 -> Binary Logic4/2
  Extract5/1 -> Binary Logic5/1
  Extract35/1 -> Binary Logic5/2
  Extract6/1 -> Binary Logic6/1
  Extract36/1 -> Binary Logic6/2
  Extract7/1 -> Binary Logic7/1
  Extract37/1 -> Binary Logic7/2
  Extract8/1 -> Binary Logic8/1
  Extract38/1 -> Binary Logic8/2
  Extract9/1 -> Binary Logic9/1
  Extract39/1 -> Binary Logic9/2
  Extract22/1 -> Binary Logic10/2
  Extract10/1 -> Binary Logic10/1
  Extract23/1 -> Binary Logic11/2
  Extract11/1 -> Binary Logic11/1
  Extract12/1 -> Binary Logic12/1
  Extract24/1 -> Binary Logic12/2
  Extract13/1 -> Binary Logic13/1
  Extract25/1 -> Binary Logic13/2
  Extract14/1 -> Binary Logic14/1
  Extract26/1 -> Binary Logic14/2
  Extract15/1 -> Binary Logic15/1
  Extract27/1 -> Binary Logic15/2
  Binary Logic7/1 -> Concat1/4
  Binary Logic6/1 -> Concat1/3
  Binary Logic5/1 -> Concat1/2
  Binary Logic4/1 -> Concat1/1
  Binary Logic3/1 -> Concat/4
  Binary Logic2/1 -> Concat/3
  Binary Logic1/1 -> Concat/2
  Binary Logic/1 -> Concat/1
  Binary Logic15/1 -> Concat2/1
  Binary Logic14/1 -> Concat2/2
  Binary Logic13/1 -> Concat2/3
  Binary Logic12/1 -> Concat2/4
  Binary Logic11/1 -> Concat3/1
  Binary Logic10/1 -> Concat3/2
  Binary Logic9/1 -> Concat3/3
  Binary Logic8/1 -> Concat3/4
  Concat/1 -> Out1/1
  Concat1/1 -> Out2/1
  Concat2/1 -> Out3/1
  Concat3/1 -> Out4/1
